simulink model "option1"  (R2023b)
settings: Solver=VariableStepAuto  StartTime=0.0  StopTime=10.0  RelTol=1e-3
values from neighbouring files (symbols this model uses):
  b1 = 1    [combined_options_code.m]    (also in option1_code.m; option2_code.m; option3_code.m)
  b2 = 1    [combined_options_code.m]    (also in option1_code.m; option2_code.m; option3_code.m)
  J1 = 100    [combined_options_code.m]    (also in option1_code.m; option2_code.m; option3_code.m)
  J2 = 1    [combined_options_code.m]    (also in option1_code.m; option2_code.m; option3_code.m)
  stiffness = k_values(k)    [combined_options_code.m]    (also in option1_code.m)
  torque_iteration = A_constant_torque_S1(x)    [combined_options_code.m]    (also in option1_code.m; option2_code.m; option3_code.m)
  torque_iteration2 = A_constant_torque_S2(x)    [combined_options_code.m]    (also in option1_code.m; option2_code.m; option3_code.m)
settings Model: Creator=Conor  LastModifiedBy=Conor

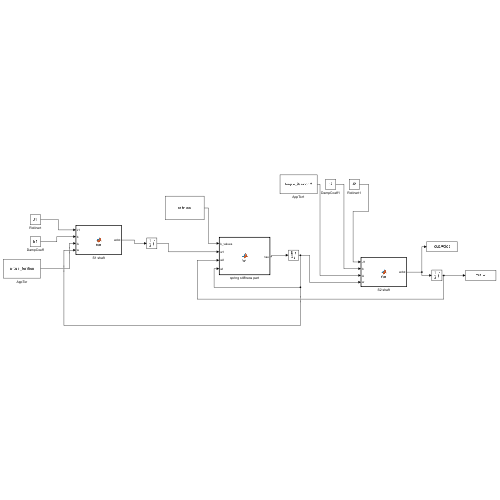
[thumbnail: Simulink's stored preview of the top-level diagram]
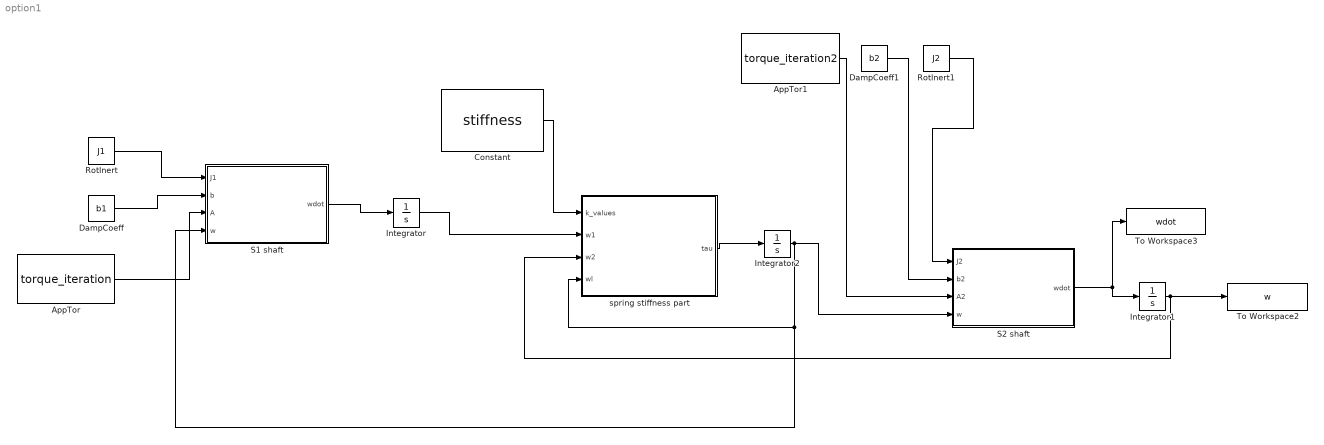
== system option1 ==
  AppTor : Constant  Value=torque_iteration
  AppTor1 : Constant  Value=torque_iteration2
  Constant : Constant  Value=stiffness
  DampCoeff : Constant  Value=b1
  DampCoeff1 : Constant  Value=b2
  Integrator : Integrator  LimitOutput=on  UpperSaturationLimit=10
  Integrator1 : Integrator  LimitOutput=on  UpperSaturationLimit=10
  Integrator2 : Integrator  LimitOutput=on  UpperSaturationLimit=10
  RotInert : Constant  Value=J1  SampleTime=-1
  RotInert1 : Constant  Value=J2  SampleTime=-1
  S1 shaft : MATLAB Function  TreatAsAtomicUnit=on
  S2 shaft : MATLAB Function  TreatAsAtomicUnit=on
  To Workspace2 : ToWorkspace  VariableName=w  SaveFormat=Timeseries  SampleTime=-1
  To Workspace3 : ToWorkspace  VariableName=wdot  SaveFormat=Timeseries  SampleTime=-1
  spring stiffness part : MATLAB Function  TreatAsAtomicUnit=on
  wires:
  Integrator/1 -> spring stiffness part/2(w1)
  RotInert/1 -> S1 shaft/1(J1)
  AppTor/1 -> S1 shaft/3(A)
  DampCoeff/1 -> S1 shaft/2(b)
  S1 shaft/1(wdot) -> Integrator/1
  S2 shaft/1(wdot) -> To Workspace3/1, Integrator1/1
  AppTor1/1 -> S2 shaft/3(A2)
  DampCoeff1/1 -> S2 shaft/2(b2)
  RotInert1/1 -> S2 shaft/1(J2)
  Integrator1/1 -> spring stiffness part/3(w2), To Workspace2/1
  Constant/1 -> spring stiffness part/1(k_values)
  spring stiffness part/1(tau) -> Integrator2/1
  Integrator2/1 -> spring stiffness part/4(wl), S1 shaft/4(w), S2 shaft/4(w)

== matlab function option1/S2 shaft ==
  data: J2 input; wdot output; b2 input; A2 input; w input
function wdot = fcn(J2, b2, A2, w)

wdot = (1 / J2) * (A2 - b2*w);

== matlab function option1/S1 shaft ==
  data: J1 input; wdot output; b input; A input; w input
function wdot = fcn(J1, b, A, w)

wdot = (1 / J1) * (A - b*w);

== matlab function option1/spring stiffness part ==
  data: k_values input; w1 input; tau output; w2 input; wl input
function tau = fcn(k_values, w1, w2, wl)

tau = k_values*(w1 - w2 - wl);
